simulink model "torque_calcs"  (R2024b)
settings: Solver=FixedStepAuto  StartTime=0.0  StopTime=10  FixedStep=0.01  RelTol=1e-3
values from neighbouring files (symbols this model uses):
  damping_force = zeros(size(vel_range))    [model_params.m]
  M_cart = 0.5    [model_params.m]
  R_crank = 1 / 39.37    (= 0.0254000508001)    [model_params.m]
  theta_dot_const = max_linear_speed / R_crank    (= 5)    [model_params.m]
  vel_range = linspace(-max_linear_speed, max_linear_speed, 50)    [model_params.m]
undefined symbols (not defined in the file or in its folder): theta0_dot
settings Model: Creator=lucas  LastModifiedBy=lucas

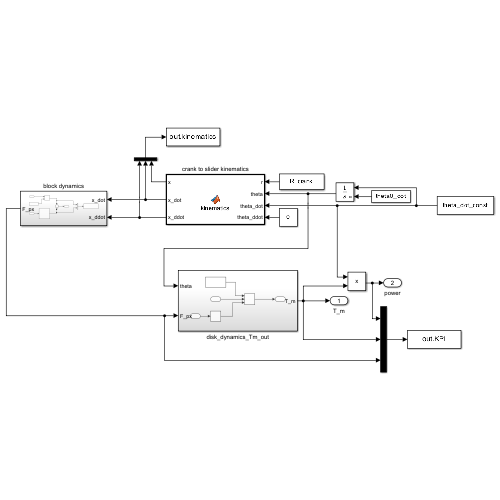
[thumbnail: Simulink's stored preview of the top-level diagram]
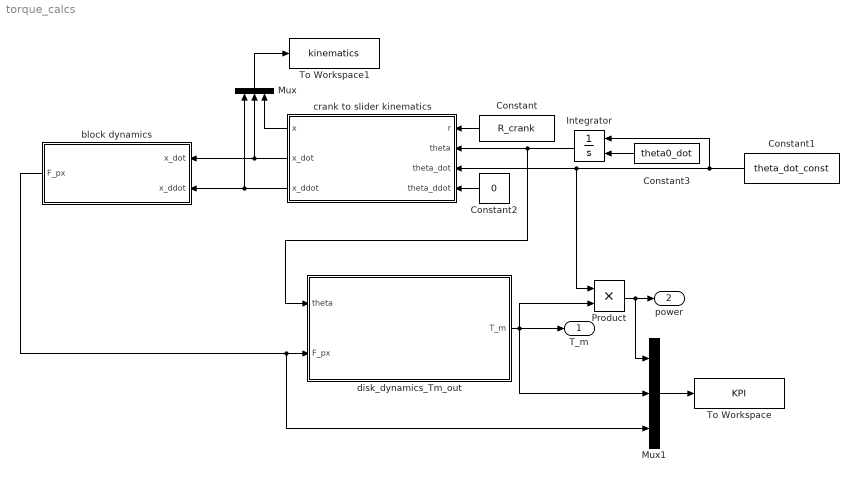
== system torque_calcs ==
  Constant : Constant  Value=R_crank
  Constant1 : Constant  Value=theta_dot_const
  Constant2 : Constant  Value=0
  Constant3 : Constant  Value=theta0_dot
  Integrator : Integrator  InitialConditionSource=external
  Mux : Mux  Inputs=3
  Mux1 : Mux  Inputs=3
  Product : Product
  To Workspace : ToWorkspace  VariableName=KPI  SaveFormat=Structure With Time  SampleTime=-1
  To Workspace1 : ToWorkspace  VariableName=kinematics  SaveFormat=Timeseries  SampleTime=-1
  block dynamics : Subsystem
  crank to slider kinematics : MATLAB Function  TreatAsAtomicUnit=on
  disk_dynamics_Tm_out : Subsystem
  T_m : Outport
  power : Outport  Port=2
  wires:
  Constant/1 -> crank to slider kinematics/1(r)
  crank to slider kinematics/2(x_dot) -> block dynamics/1(x_dot), Mux/2
  crank to slider kinematics/3(x_ddot) -> block dynamics/2(x_ddot), Mux/1
  block dynamics/1(F_px) -> Mux1/3, disk_dynamics_Tm_out/2(F_px)
  disk_dynamics_Tm_out/1(T_m) -> Mux1/2, Product/2, T_m/1
  Integrator/1 -> disk_dynamics_Tm_out/1(theta), crank to slider kinematics/2(theta)
  Constant2/1 -> crank to slider kinematics/4(theta_ddot)
  Constant3/1 -> Integrator/2
  Constant1/1 -> crank to slider kinematics/3(theta_dot), Product/1, Integrator/1
  Product/1 -> Mux1/1, power/1
  crank to slider kinematics/1(x) -> Mux/3
  Mux1/1 -> To Workspace/1
  Mux/1 -> To Workspace1/1

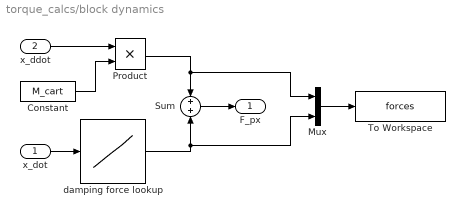
== system torque_calcs/block dynamics ==
  x_dot : Inport
  x_ddot : Inport  Port=2
  Constant : Constant  Value=M_cart
  Mux : Mux  Inputs=2
  Product : Product
  Sum : Sum  Inputs=+|+
  To Workspace : ToWorkspace  VariableName=forces  SaveFormat=Structure With Time  SampleTime=-1
  damping force lookup : Lookup_n-D  NumberOfTableDimensions=1  BreakpointsForDimension1=vel_range  Table=damping_force  InternalRulePriority=Speed  RndMeth=Simplest
  F_px : Outport
  wires:
  x_ddot/1 -> Product/1
  Constant/1 -> Product/2
  x_dot/1 -> damping force lookup/1
  Product/1 -> Mux/1, Sum/1
  damping force lookup/1 -> Mux/2, Sum/2
  Sum/1 -> F_px/1
  Mux/1 -> To Workspace/1

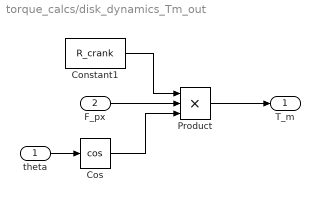
== system torque_calcs/disk_dynamics_Tm_out ==
  theta : Inport
  F_px : Inport  Port=2
  Constant1 : Constant  Value=R_crank
  Cos : Trigonometry  Operator=cos
  Product : Product  Inputs=3
  T_m : Outport
  wires:
  theta/1 -> Cos/1
  Constant1/1 -> Product/1
  F_px/1 -> Product/2
  Cos/1 -> Product/3
  Product/1 -> T_m/1

== matlab function torque_calcs/crank to slider kinematics ==
  data: r input; x output; theta input; theta_dot input; theta_ddot input; x_dot output; x_ddot output
function [x, x_dot, x_ddot] = kinematics(r, theta, theta_dot, theta_ddot)

x = r * sin(theta);
x_dot = r * theta_dot*cos(theta);
x_ddot = r*(theta_ddot * cos(theta) - theta_dot^2 * sin(theta));

end
